simulink model "VVI_group11"  (R2023a)
settings: Solver=FixedStepAuto  StartTime=0.0  StopTime=10.0  FixedStep=1e-3  RelTol=1e-3  EnableMultiTasking=on
undefined symbols (not defined in the file): D1, D10, D12, D13, D2, D3, D5, D7, D9, PTA1, PTA2, PTB9, PTC17, PTC3, PTC4, PTD0, PTD1, PTD3
libraries: frdmk64flib x11
settings Model: ExtModeTrigDuration=5  Creator=faraa  LastModifiedBy=faraa
settings OptimizationCC: EnhancedBackFolding=on  PassReuseOutputArgsAs=Individual arguments  ZeroExternalMemoryAtStartup=off  ZeroInternalMemoryAtStartup=off  MaxStackSize=64  OptimizeBlockOrder=speed  DifferentSizesBufferReuse=on  OptimizationCustomize=off  EfficientTunableParamExpr=on
settings DebuggingCC: ParameterTunabilityLossMsg=error
settings HardwareCC: ProdBitPerPointer=32  ProdBitPerSizeT=32  ProdBitPerPtrDiffT=32  ProdLargestAtomicInteger=Long  ProdLargestAtomicFloat=Double  ProdWordSize=32  ProdHWDeviceType=ARM Compatible->ARM Cortex
settings SFSimCC: MATLABDynamicMemAlloc=off
settings RTWCC: Description=Embedded Coder  SystemTargetFile=ert.tlc  HardwareBoard=NXP FRDM-K64F  TLCOptions="-aInlineSetEventsForThisBaseRateFcn=TLC_FALSE -aSuppressMultiTaskScheduler=TLC_FALSE  -aRateBasedStepFcn=0"  TemplateMakefile=ert_default_tmf  Toolchain=GNU Tools for ARM Embedded Processors
settings CodeAppCC: ForceParamTrailComments=on  IgnoreCustomStorageClasses=off  OperatorAnnotations=on  SimulinkDataObjDesc=on  SFDataObjDesc=on  InsertBlockDesc=on
settings ERTTargetCC: ExtModeTransport=4  ExtModeMexFile=sendToCommService

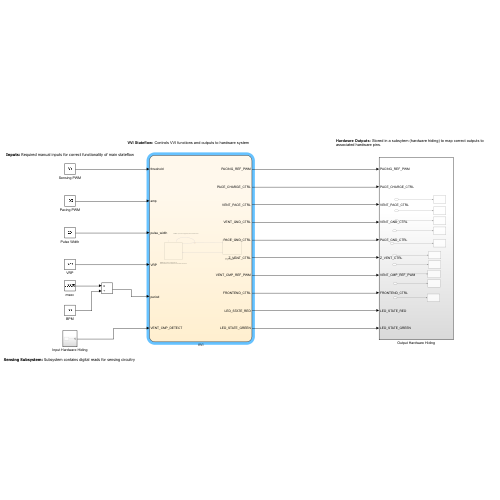
[thumbnail: Simulink's stored preview of the top-level diagram]
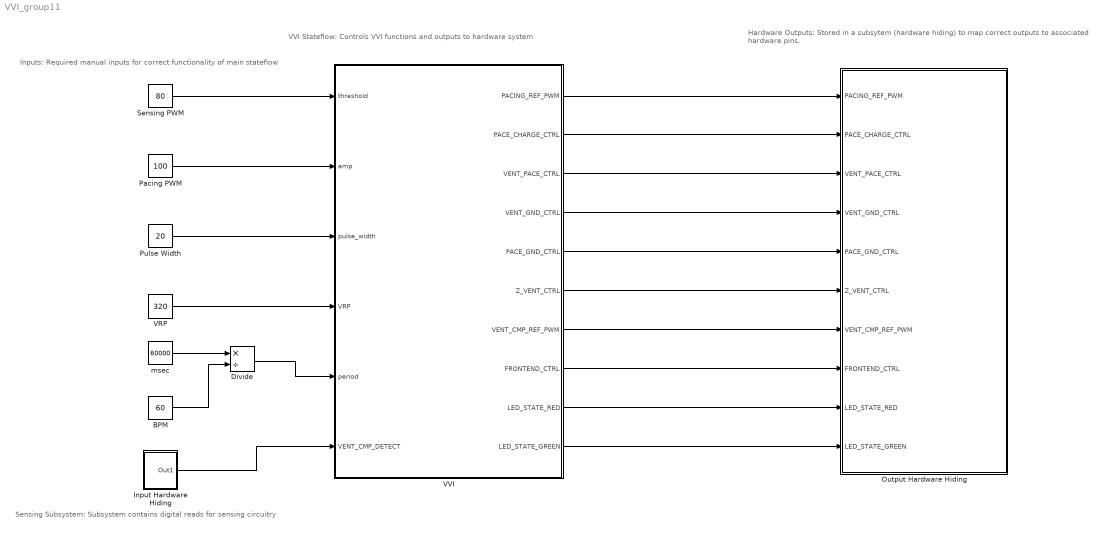
== system VVI_group11 ==
  note: Sensing Subsystem: Subsystem contains digital reads for sensing circuitry
  note: Inputs: Required manual inputs for correct functionality of main stateflow
  note: VVI Stateflow: Controls VVI functions and outputs to hardware system
  note: Hardware Outputs: Stored in a subsytem (hardware hiding) to map correct outputs to associated hardware pins.
  BPM : Constant  Value=60
  Divide : Product  Inputs=*/
  Input Hardware Hiding : Subsystem
  Output Hardware Hiding : Subsystem
  Pacing PWM : Constant  Value=100
  Pulse Width : Constant  Value=20
  Sensing PWM : Constant  Value=80
  VRP : Constant  Value=320
  VVI : Stateflow chart  TreatAsAtomicUnit=on
  msec : Constant  Value=60000
  wires:
  VVI/10(LED_STATE_GREEN) -> Output Hardware Hiding/10(LED_STATE_GREEN)
  VVI/3(VENT_PACE_CTRL) -> Output Hardware Hiding/3(VENT_PACE_CTRL)
  VVI/6(Z_VENT_CTRL) -> Output Hardware Hiding/6(Z_VENT_CTRL)
  VVI/7(VENT_CMP_REF_PWM) -> Output Hardware Hiding/7(VENT_CMP_REF_PWM)
  VVI/1(PACING_REF_PWM) -> Output Hardware Hiding/1(PACING_REF_PWM)
  VVI/9(LED_STATE_RED) -> Output Hardware Hiding/9(LED_STATE_RED)
  Pacing PWM/1 -> VVI/2(amp)
  VVI/2(PACE_CHARGE_CTRL) -> Output Hardware Hiding/2(PACE_CHARGE_CTRL)
  VVI/5(PACE_GND_CTRL) -> Output Hardware Hiding/5(PACE_GND_CTRL)
  VVI/4(VENT_GND_CTRL) -> Output Hardware Hiding/4(VENT_GND_CTRL)
  Input Hardware Hiding/1(Out1) -> VVI/6(VENT_CMP_DETECT)
  Pulse Width/1 -> VVI/3(pulse_width)
  VVI/8(FRONTEND_CTRL) -> Output Hardware Hiding/8(FRONTEND_CTRL)
  Divide/1 -> VVI/5(period)
  BPM/1 -> Divide/2
  msec/1 -> Divide/1
  Sensing PWM/1 -> VVI/1(threshold)
  VRP/1 -> VVI/4(VRP)

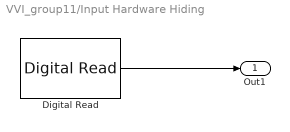
== system VVI_group11/Input Hardware Hiding ==
  Digital Read : frdmk64flib/Digital Read  Whichpin=PTC17 (D1)  SampleTime=-1
  Out1 : Outport
  wires:
  Digital Read/1 -> Out1/1

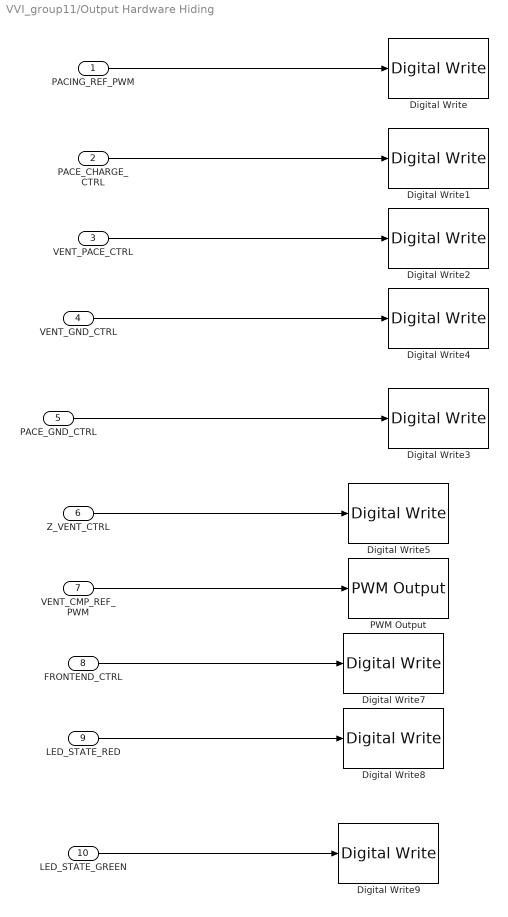
== system VVI_group11/Output Hardware Hiding ==
  PACING_REF_PWM : Inport
  PACE_CHARGE_CTRL : Inport  Port=2
  VENT_PACE_CTRL : Inport  Port=3
  VENT_GND_CTRL : Inport  Port=4
  PACE_GND_CTRL : Inport  Port=5
  Z_VENT_CTRL : Inport  Port=6
  VENT_CMP_REF_PWM : Inport  Port=7
  FRONTEND_CTRL : Inport  Port=8
  LED_STATE_RED : Inport  Port=9
  LED_STATE_GREEN : Inport  Port=10
  Digital Write : frdmk64flib/Digital Write  Whichpin=PTA2 (D5)
  Digital Write1 : frdmk64flib/Digital Write  Whichpin=PTB9 (D2)
  Digital Write2 : frdmk64flib/Digital Write  Whichpin=PTC4 (D9)
  Digital Write3 : frdmk64flib/Digital Write  Whichpin=PTD0 (D10)
  Digital Write4 : frdmk64flib/Digital Write  Whichpin=PTD3 (D12)
  Digital Write5 : frdmk64flib/Digital Write  Whichpin=PTC3 (D7)
  Digital Write7 : frdmk64flib/Digital Write  Whichpin=PTD1 (D13)
  Digital Write8 : frdmk64flib/Digital Write  Whichpin=RED_LED
  Digital Write9 : frdmk64flib/Digital Write  Whichpin=GREEN_LED
  PWM Output : frdmk64flib/PWM Output  Whichpin=PTA1 (D3)  InitialFrequency=2000  InitialDutyCycle=0
  wires:
  PACING_REF_PWM/1 -> Digital Write/1
  PACE_CHARGE_CTRL/1 -> Digital Write1/1
  VENT_PACE_CTRL/1 -> Digital Write2/1
  PACE_GND_CTRL/1 -> Digital Write3/1
  VENT_GND_CTRL/1 -> Digital Write4/1
  Z_VENT_CTRL/1 -> Digital Write5/1
  VENT_CMP_REF_PWM/1 -> PWM Output/1
  FRONTEND_CTRL/1 -> Digital Write7/1
  LED_STATE_RED/1 -> Digital Write8/1
  LED_STATE_GREEN/1 -> Digital Write9/1

== stateflow chart VVI_group11/VVI ==
  note: Condition: Loops back to charging/sensing based on threshold detection
  state Pacing
    entry:
    PACING_REF_PWM = amp;
    PACE_CHARGE_CTRL = 0;
    VENT_PACE_CTRL = 1;
    VENT_GND_CTRL =0;
    PACE_GND_CTRL = 1;
    Z_VENT_CTRL =0;
    LED_STATE_RED = false;
    LED_STATE_GREEN = true;
    FRONTEND_CTRL = 1;
  state Charging_Sensing
    %CHARGING
    entry:
    PACING_REF_PWM = amp;
    PACE_CHARGE_CTRL = 1;
    VENT_PACE_CTRL = 0;
    VENT_GND_CTRL =1;
    PACE_GND_CTRL = 0;
    Z_VENT_CTRL = 0;
    %sSENSING
    FRONTEND_CTRL = 1;
    VENT_CMP_REF_PWM = threshold;
    LED_STATE_RED = true;
    LED_STATE_GREEN = false;
  note: Pacing: Discharges C22 and charges C21
      | and triggers LED indicators
  note: Charging: State to Charge C22 and discharge C21,
      | trigger LED indicators as well as implement sensing to determine when to pulse
  (junction 31) -> Charging_Sensing [order 1] : [VENT_CMP_DETECT == 1]
  (default) -> Charging_Sensing
  (junction 31) -> Pacing [order 2] : after(period-pulse_width,msec)[VENT_CMP_DETECT == 0]
  Charging_Sensing -> (junction 31) : [after(VRP-pulse_width,msec)]
  Pacing -> Charging_Sensing : [after(pulse_width,msec)]
  data: threshold input; amp input; pulse_width input; VRP input; period input; VENT_CMP_DETECT input; PACING_REF_PWM output; PACE_CHARGE_CTRL output; VENT_PACE_CTRL output; VENT_GND_CTRL output; PACE_GND_CTRL output; Z_VENT_CTRL output; VENT_CMP_REF_PWM output; FRONTEND_CTRL output; LED_STATE_RED output; LED_STATE_GREEN output
